simulink model "ReducingofBlockDiagram"  (R2018a)
settings: Solver=VariableStepAuto  StartTime=0.0  StopTime=10.0  RelTol=1e-3
undefined symbols (not defined in the file): fm, fmkm, Jm, km, La, LaJm, Ra, Rafmkm, sJm, sLa
settings Model: Creator=Neo  LastModifiedBy=Neo

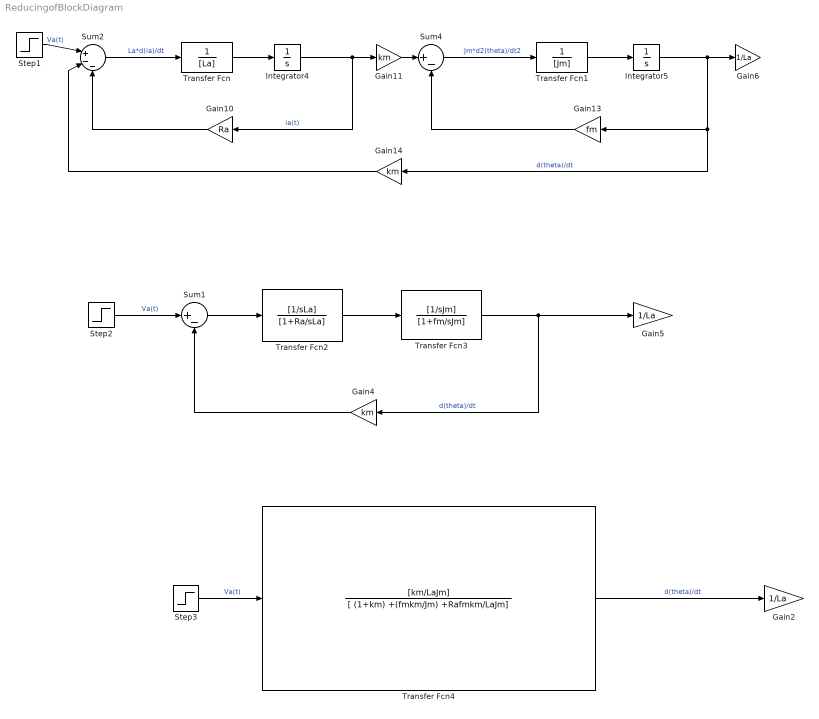
== system ReducingofBlockDiagram ==
  Gain10 : Gain  Gain=Ra
  Gain11 : Gain  Gain=km
  Gain13 : Gain  Gain=fm
  Gain14 : Gain  Gain=km
  Gain2 : Gain  Gain=1/La
  Gain4 : Gain  Gain=km
  Gain5 : Gain  Gain=1/La
  Gain6 : Gain  Gain=1/La
  Integrator4 : Integrator
  Integrator5 : Integrator
  Step1 : Step  Time=0  After=10  SampleTime=0
  Step2 : Step  Time=0  After=10  SampleTime=0
  Step3 : Step  Time=0  After=10  SampleTime=0
  Sum1 : Sum  Inputs=|+-
  Sum2 : Sum  Inputs=|+--
  Sum4 : Sum  Inputs=|+-
  Transfer Fcn : TransferFcn  Denominator=[La]
  Transfer Fcn1 : TransferFcn  Denominator=[Jm]
  Transfer Fcn2 : TransferFcn  Numerator=[1/sLa]  Denominator=[1+Ra/sLa]
  Transfer Fcn3 : TransferFcn  Numerator=[1/sJm]  Denominator=[1+fm/sJm]
  Transfer Fcn4 : TransferFcn  Numerator=[km/LaJm]  Denominator=[ (1+km) +(fmkm/Jm) +Rafmkm/LaJm]
  wires:
  Gain14/1 -> Sum2/2
  Step1/1 -> Sum2/1  "Va(t)"
  Gain13/1 -> Sum4/2
  Gain11/1 -> Sum4/1
  Integrator5/1 -> Gain13/1, Gain14/1, Gain6/1  "d(theta)/dt"
  Gain10/1 -> Sum2/3
  Integrator4/1 -> Gain11/1, Gain10/1  "ia(t)"
  Gain4/1 -> Sum1/2
  Step2/1 -> Sum1/1  "Va(t)"
  Sum2/1 -> Transfer Fcn/1  "La*d(ia)/dt"
  Transfer Fcn/1 -> Integrator4/1
  Sum4/1 -> Transfer Fcn1/1  "Jm*d2(theta)/dt2"
  Transfer Fcn1/1 -> Integrator5/1
  Sum1/1 -> Transfer Fcn2/1
  Transfer Fcn2/1 -> Transfer Fcn3/1
  Transfer Fcn3/1 -> Gain5/1, Gain4/1  "d(theta)/dt"
  Step3/1 -> Transfer Fcn4/1  "Va(t)"
  Transfer Fcn4/1 -> Gain2/1  "d(theta)/dt"
